simulink model "projektlodowisko"  (R2015a)
settings: Solver=ode45  StartTime=0.0  StopTime=4000  RelTol=1e-3
undefined symbols (not defined in the file or in its folder): sigbuilder_block
libraries: simulink x1
settings Model: Creator=346  LastModifiedBy=lenovo

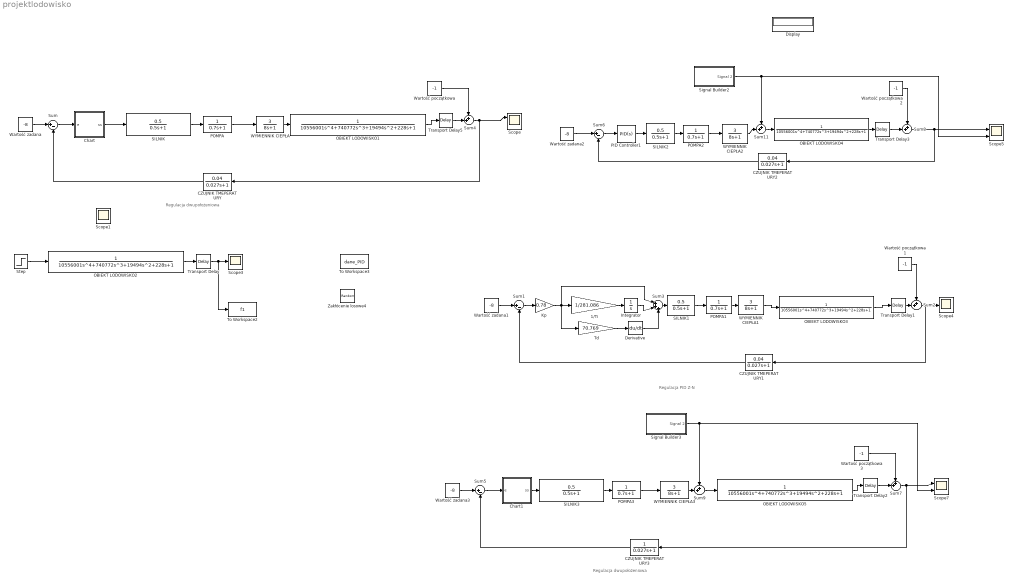
== system projektlodowisko ==
  note: Regulacja dwupołożeniowa
  note: Regulacja PID Z-N
  note: Regulacja dwupołożeniowa
  1/Ti : Gain  Gain=1/281.086
  CZUJNIK TMEPERATURY : TransferFcn  Numerator=[0.04]  Denominator=[0.027 1]
  CZUJNIK TMEPERATURY1 : TransferFcn  Numerator=[0.04]  Denominator=[0.027 1]
  CZUJNIK TMEPERATURY2 : TransferFcn  Numerator=[0.04]  Denominator=[0.027 1]
  CZUJNIK TMEPERATURY3 : TransferFcn  Denominator=[0.027 1]
  Chart : Stateflow chart  TreatAsAtomicUnit=on
  Chart1 : Stateflow chart  TreatAsAtomicUnit=on
  Derivative : Derivative
  Display : Display
  Integrator : Integrator
  Kp : Gain  Gain=0.78
  OBIEKT LODOWISKO1 : TransferFcn  Denominator=[ 10556001 740772 19494 228 1]
  OBIEKT LODOWISKO2 : TransferFcn  Denominator=[10556001 740772 19494 228 1]
  OBIEKT LODOWISKO3 : TransferFcn  Denominator=[10556001 740772 19494 228 1]
  OBIEKT LODOWISKO4 : TransferFcn  Denominator=[10556001 740772 19494 228 1]
  OBIEKT LODOWISKO5 : TransferFcn  Denominator=[ 10556001 740772 19494 228 1]
  PID Controller1 : simulink/Continuous/PID Controller  Controller=PID  TimeDomain=Continuous-time  SampleTime=-1  IntegratorMethod=Forward Euler  FilterMethod=Forward Euler  Form=Parallel  UseFilter=on  ControllerParametersSource=internal  P=0.233912329939403  I=0.00168979130879857  D=0  N=100  InitialConditionSource=internal  InitialConditionForIntegrator=0  InitialConditionForFilter=0  ExternalReset=none  LimitOutput=off  UpperSaturationLimit=inf  LowerSaturationLimit=-inf  LinearizeAsGain=on  AntiWindupMode=none  Kb=1  TrackingMode=off  Kt=1  PParamMin=[]  PParamMax=[]  IParamMin=[]  IParamMax=[]  DParamMin=[]  DParamMax=[]  NParamMin=[]  NParamMax=[]  KbParamMin=[]  KbParamMax=[]  KtParamMin=[]  KtParamMax=[]  POutMin=[]  POutMax=[]  IOutMin=[]  IOutMax=[]  DOutMin=[]  DOutMax=[]  NOutMin=[]  NOutMax=[]  KbOutMin=[]  KbOutMax=[]  KtOutMin=[]  KtOutMax=[]  IntegratorOutMin=[]  IntegratorOutMax=[]  FilterOutMin=[]  FilterOutMax=[]  SumOutMin=[]  SumOutMax=[]  SumI1OutMin=[]  SumI1OutMax=[]  SumI2OutMin=[]  SumI2OutMax=[]  SumI3OutMin=[]  SumI3OutMax=[]  SumDOutMin=[]  SumDOutMax=[]  SaturationOutMin=[]  SaturationOutMax=[]  IntegratorContinuousStateAttributes=''  IntegratorStateMustResolveToSignalObject=off  IntegratorRTWStateStorageClass=Auto  FilterContinuousStateAttributes=''  FilterStateMustResolveToSignalObject=off  FilterRTWStateStorageClass=Auto  DifferentiatorICPrevScaledInput=0  DifferentiatorOutMin=[]  DifferentiatorOutMax=[]
  POMPA{,1..3} (4 alike) : TransferFcn  Denominator=[ 0.7 1]
  SILNIK{,1..3} (4 alike) : TransferFcn  Numerator=[0.5]  Denominator=[ 0.5 1]
  Scope : Scope  NumInputPorts=2
      settings: TimeRange=4000  YMin=-10~-5  YMax=-1~5
  Scope1 : Scope
      settings: YMin=-1  YMax=2
  Scope3 : Scope
      settings: YMin=-1  YMax=2  SaveName=ScopeData3
  Scope4 : Scope
      settings: TimeRange=2000  YMin=-7.8  YMax=-5.4  SaveName=ScopeData4
  Scope5 : Scope  NumInputPorts=2
      settings: TimeRange=4000  YMin=-8.4~-5  YMax=-7.55~5  SaveName=ScopeData5
  Scope7 : Scope  NumInputPorts=2
      settings: TimeRange=5000  YMin=-10.25~-5  YMax=-5.75~5  SaveName=ScopeData7
  Signal Builder2 : Subsystem  Tag=STV Subsys  LoadFcn=sigbuilder_block('load');  StartFcn=sigbuilder_block('start');  StopFcn=sigbuilder_block('stop');  ClipboardFcn=sigbuilder_block('clipboard');  mask(Sigbuilder block){}
      mask help: Simulink:masks:SigbuilderBlock_MD
      mask init:
      | if ~strcmp(get_param(bdroot(gcbh),'SimulationStatus'),'stopped') tuvar = sigbuilder_block('maskInit'); end
      settings: CopyFcn=sigbuilder_block('copy');  DeleteFcn=sigbuilder_block('delete');  ModelCloseFcn=sigbuilder_block('modelClose');  PreSaveFcn=sigbuilder_block('preSave');  PauseFcn=sigbuilder_block('pause');  ContinueFcn=sigbuilder_block('continue');  NameChangeFcn=sigbuilder_block('namechange');  OpenFcn=sigbuilder_block('open',[437.6 199.2 550.4 400 ]);  CloseFcn=sigbuilder_block('close');
      mask Display: plot(0, 0, 100, 100,[2, 2, 32, 32, 2], [68, 8, 8, 68, 68],[32, 2], [38, 38], [32, 19, 2],[53, 60, 44], [32, 17, 17, 2],[16, 16, 31, 31]);txt = getActiveGroup(gcbh);text(2, 100, txt,'verticalAlignment', 'top');
  Signal Builder3 : Subsystem  Tag=STV Subsys  LoadFcn=sigbuilder_block('load');  StartFcn=sigbuilder_block('start');  StopFcn=sigbuilder_block('stop');  ClipboardFcn=sigbuilder_block('clipboard');  mask(Sigbuilder block){}
      mask help: Simulink:masks:SigbuilderBlock_MD
      mask init:
      | if ~strcmp(get_param(bdroot(gcbh),'SimulationStatus'),'stopped') tuvar = sigbuilder_block('maskInit'); end
      settings: CopyFcn=sigbuilder_block('copy');  DeleteFcn=sigbuilder_block('delete');  ModelCloseFcn=sigbuilder_block('modelClose');  PreSaveFcn=sigbuilder_block('preSave');  PauseFcn=sigbuilder_block('pause');  ContinueFcn=sigbuilder_block('continue');  NameChangeFcn=sigbuilder_block('namechange');  OpenFcn=sigbuilder_block('open',[437.6 199.2 550.4 400 ]);  CloseFcn=sigbuilder_block('close');
      mask Display: plot(0, 0, 100, 100,[2, 2, 32, 32, 2], [68, 8, 8, 68, 68],[32, 2], [38, 38], [32, 19, 2],[53, 60, 44], [32, 17, 17, 2],[16, 16, 31, 31]);txt = getActiveGroup(gcbh);text(2, 100, txt,'verticalAlignment', 'top');
  Step : Step  SampleTime=0
  Sum{,1,5..6} (4 alike) : Sum  Inputs=|+-
  Sum{2,4,7..9,11} (6 alike) : Sum  Inputs=++|
  Sum3 : Sum  Inputs=|+++
  Td : Gain  Gain=70.769
  To Workspace2 : ToWorkspace  VariableName=f1  SaveFormat=Timeseries  SampleTime=-1
  To Workspace3 : ToWorkspace  VariableName=dane_PID  SaveFormat=Timeseries  SampleTime=-1
  Transport Delay : TransportDelay  DelayTime=60
  Transport Delay{1..3,5} (4 alike) : TransportDelay  DelayTime=70
  WYMIENNIK CIEPŁA{,1..3} (4 alike) : TransferFcn  Numerator=[3]  Denominator=[ 8 1]
  Wartość początkowa{,1..3} (4 alike) : Constant  Value=-1
  Wartość zadana{,1..3} (4 alike) : Constant  Value=-8
  Zakłócenie losowe4 : RandomNumber  Mean=0.2  Variance=0.3  SampleTime=70
  wires:
  Wartość zadana/1 -> Sum/1
  SILNIK/1 -> POMPA/1
  POMPA/1 -> WYMIENNIK CIEPŁA/1
  CZUJNIK TMEPERATURY/1 -> Sum/2
  Sum/1 -> Chart/1(e)
  Wartość początkowa/1 -> Sum4/1
  Step/1 -> OBIEKT LODOWISKO2/1
  OBIEKT LODOWISKO2/1 -> Transport Delay/1
  Transport Delay/1 -> To Workspace2/1, Scope3/1
  SILNIK2/1 -> POMPA2/1
  POMPA2/1 -> WYMIENNIK CIEPŁA2/1
  CZUJNIK TMEPERATURY2/1 -> Sum6/2
  Sum8/1 -> Scope5/1, CZUJNIK TMEPERATURY2/1
  Wartość początkowa2/1 -> Sum8/1
  OBIEKT LODOWISKO4/1 -> Transport Delay3/1
  Transport Delay3/1 -> Sum8/2
  Wartość zadana2/1 -> Sum6/1
  Sum4/1 -> CZUJNIK TMEPERATURY/1, Scope/1
  WYMIENNIK CIEPŁA/1 -> OBIEKT LODOWISKO1/1
  SILNIK1/1 -> POMPA1/1
  POMPA1/1 -> WYMIENNIK CIEPŁA1/1
  CZUJNIK TMEPERATURY1/1 -> Sum1/2
  Sum2/1 -> Scope4/1, CZUJNIK TMEPERATURY1/1
  Wartość początkowa1/1 -> Sum2/1
  OBIEKT LODOWISKO3/1 -> Transport Delay1/1
  Transport Delay1/1 -> Sum2/2
  Wartość zadana1/1 -> Sum1/1
  1/Ti/1 -> Integrator/1
  Kp/1 -> 1/Ti/1, Td/1, Sum3/1
  Td/1 -> Derivative/1
  Derivative/1 -> Sum3/3
  Integrator/1 -> Sum3/2
  Sum3/1 -> SILNIK1/1
  Wartość zadana3/1 -> Sum5/1
  SILNIK3/1 -> POMPA3/1
  POMPA3/1 -> WYMIENNIK CIEPŁA3/1
  CZUJNIK TMEPERATURY3/1 -> Sum5/2
  Sum5/1 -> Chart1/1(e)
  Wartość początkowa3/1 -> Sum7/1
  Sum7/1 -> Scope7/1, CZUJNIK TMEPERATURY3/1
  Chart1/1(ss) -> SILNIK3/1
  Transport Delay2/1 -> Sum7/2
  OBIEKT LODOWISKO5/1 -> Transport Delay2/1
  WYMIENNIK CIEPŁA3/1 -> Sum9/2
  Sum9/1 -> OBIEKT LODOWISKO5/1
  Signal Builder3/1(Signal 2) -> Sum9/1, Scope7/2
  PID Controller1/1 -> SILNIK2/1
  WYMIENNIK CIEPŁA2/1 -> Sum11/2
  Sum11/1 -> OBIEKT LODOWISKO4/1
  Signal Builder2/1(Signal 2) -> Sum11/1, Scope5/2
  WYMIENNIK CIEPŁA1/1 -> OBIEKT LODOWISKO3/1
  Sum6/1 -> PID Controller1/1
  Transport Delay5/1 -> Sum4/2
  OBIEKT LODOWISKO1/1 -> Transport Delay5/1
  Chart/1(ss) -> SILNIK/1
  Sum1/1 -> Kp/1

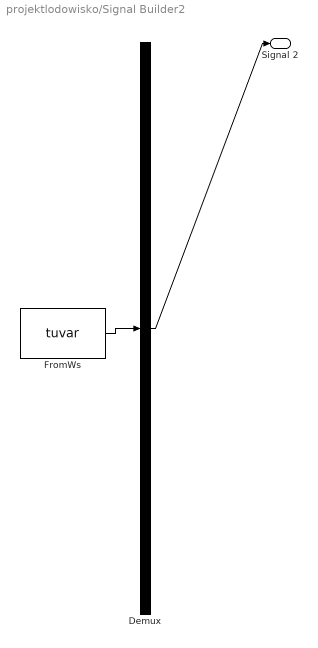
== system projektlodowisko/Signal Builder2 ==
  Demux : Demux  Tag=STV Demux  Outputs=1
  FromWs : FromWorkspace  Tag=STV FromWs  VariableName=tuvar  SampleTime=0
      SigBuilderData=|
      | common.afterFinalStr = 'Extrapolate'
      | common.sampleTime = 0
      | dataSet.timeRange = [0 5000]
      | dataSet.name = 'Group 1'
      | sbobj.Groups.Name = 'Group 1'
      | sbobj.Groups.Signals.Name = 'Signal 2'
      | sbobj.Groups.Signals.XData = [0 420 420 1050 1050 1490 1490 3125 3750 4375 5000]
      | sbobj.Groups.Signals.YData = [0.8 0.8 1.2 1.2 0.9 0.9 0.52 0.52 0.52 0.52 0.52]
      | sbobj.Groups.TimeRange = [0 5000]
  Signal 2 : Outport  Tag=STV Outport
  wires:
  FromWs/1 -> Demux/1
  Demux/1 -> Signal 2/1

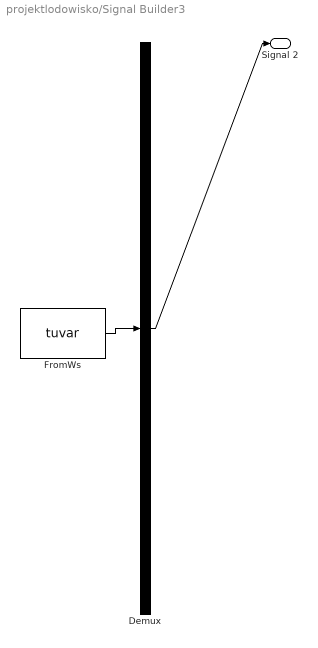
== system projektlodowisko/Signal Builder3 ==
  Demux : Demux  Tag=STV Demux  Outputs=1
  FromWs : FromWorkspace  Tag=STV FromWs  VariableName=tuvar  SampleTime=0
      SigBuilderData=|
      | common.afterFinalStr = 'Extrapolate'
      | common.sampleTime = 0
      | dataSet.timeRange = [0 5000]
      | dataSet.name = 'Group 1'
      | sbobj.Groups.Name = 'Group 1'
      | sbobj.Groups.Signals.Name = 'Signal 2'
      | sbobj.Groups.Signals.XData = [0 420 420 1050 1050 1490 1490 3125 3750 4375 5000]
      | sbobj.Groups.Signals.YData = [0.8 0.8 1.2 1.2 0.9 0.9 0.52 0.52 0.52 0.52 0.52]
      | sbobj.Groups.TimeRange = [0 5000]
  Signal 2 : Outport  Tag=STV Outport
  wires:
  FromWs/1 -> Demux/1
  Demux/1 -> Signal 2/1

== stateflow chart projektlodowisko/Chart1 ==
  state 1
    during:ss=-5.7;
  state 2
    during:ss=-3.2;
  (default) -> 1
  1 -> 2 : [e>=1]
  2 -> 1 : [e<=-1]
  data: e input; ss output

== stateflow chart projektlodowisko/Chart ==
  state 1
    during:ss=-5.6;
  state 2
    during:ss=-3.7;
  (default) -> 1
  1 -> 2 : [e>=0.7]
  2 -> 1 : [e<=-0.3]
  data: e input; ss output
